simulink model "ex_6_1"  (Simulink 10.1)
settings: Solver=VariableStepAuto  StartTime=0.0  StopTime=50  RelTol=1e-3
settings Model: Creator=Paulo Padrao  LastModifiedBy=Paulo Padrao
settings DataIOCC: SaveFormat=Dataset
settings OptimizationCC: LifeSpan=auto
settings DebuggingCC: UnderspecifiedInitializationDetection=Simplified  MergeDetectMultiDrivingBlocksExec=error  SFUnexpectedBacktrackingDiag=error  SFNoUnconditionalDefaultTransitionDiag=error  SFExecutionAtInitializationDiag=warning
settings HardwareCC: ProdBitPerPointer=64  ProdBitPerSizeT=64  ProdBitPerPtrDiffT=64  ProdLargestAtomicFloat=Float  ProdIntDivRoundTo=Zero  ProdEndianess=LittleEndian  ProdWordSize=64  ProdHWDeviceType=Intel->x86-64 (Windows64)
settings ModelReferenceCC: PropagateSignalLabelsOutOfModel=on
settings CodeAppCC: StateflowObjectComments=off
settings GRTTargetCC: TargetLangStandard=C99 (ISO)  CombineOutputUpdateFcns=on  GRTInterface=off
settings ConfigComp: CovMetricSettings=dwe  CovHtmlReporting=off  CovSaveCumulativeToWorkspaceVar=off  CovSaveSingleToWorkspaceVar=off  CovExternalEMLEnable=on

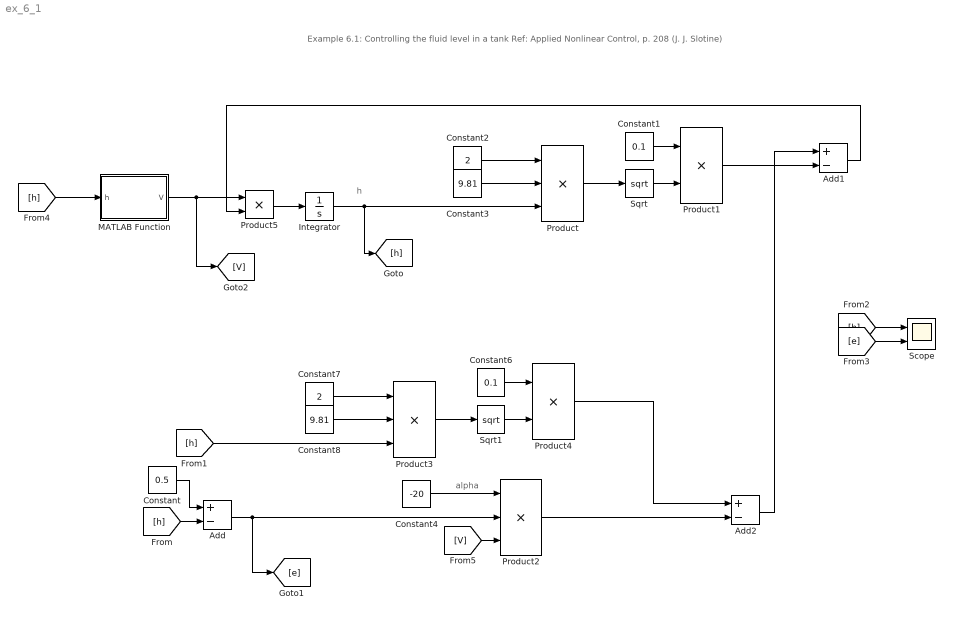
== system ex_6_1 ==
  note: Example 6.1: Controlling the fluid level in a tank
      | Ref: Applied Nonlinear Control, p. 208 (J. J. Slotine)
  note: h
  note: alpha
  Add : Sum  Inputs=+-
  Add1 : Sum  Inputs=+-
  Add2 : Sum  Inputs=+-
  Constant : Constant  Value=0.5
  Constant1 : Constant  Value=0.1
  Constant2 : Constant  Value=2
  Constant3 : Constant  Value=9.81
  Constant4 : Constant  Value=-20
  Constant6 : Constant  Value=0.1
  Constant7 : Constant  Value=2
  Constant8 : Constant  Value=9.81
  Integrator : Integrator  InitialCondition=0.1
  MATLAB Function : MATLAB Function  TreatAsAtomicUnit=on
  Product : Product  Inputs=3
  Product1 : Product
  Product2 : Product  Inputs=3
  Product3 : Product  Inputs=3
  Product4 : Product
  Product5 : Product
  Scope : Scope  NumInputPorts=2
  Sqrt : Sqrt  SaturateOnIntegerOverflow=on
  Sqrt1 : Sqrt  SaturateOnIntegerOverflow=on
  wires:
  Constant/1 -> Add/1
  Constant2/1 -> Product/1
  Constant3/1 -> Product/2
  Product/1 -> Sqrt/1
  Sqrt/1 -> Product1/2
  Constant1/1 -> Product1/1
  Constant4/1 -> Product2/1
  Integrator/1 -> [h], Product/3
  Product1/1 -> Add1/2
  [h] -> Add/2
  Add/1 -> [e], Product2/2
  Product2/1 -> Add2/2
  Product4/1 -> Add2/1
  [h] -> Product3/3
  Constant6/1 -> Product4/1
  Sqrt1/1 -> Product4/2
  Product3/1 -> Sqrt1/1
  Constant8/1 -> Product3/2
  Constant7/1 -> Product3/1
  Add2/1 -> Add1/1
  [h] -> Scope/1
  [e] -> Scope/2
  Add1/1 -> Product5/2
  Product5/1 -> Integrator/1
  MATLAB Function/1(V) -> [V], Product5/1
  [h] -> MATLAB Function/1(h)
  [V] -> Product2/3

== matlab function MATLAB Function ==
  data: h input double; V output double
function V = fcn(h)
r = 0.5;
V = pi*r*h^2 -0.33*pi*h^3;
